simulink library "mbdriLib"  (R2023b)
settings: Solver=ode45  StartTime=0.0  StopTime=10.0  RelTol=1e-3  EnableMultiTasking=on
undefined symbols (not defined in the file): ap, Newton, Raphson, uavParam
libraries: aerolibconvert2 x1, slpidlib x1, sharedtransform x1, $bdroot x1, simulink x1
settings Model: Creator=The MathWorks, Inc.  LastModifiedBy=The MathWorks, Inc.
settings SolverCC: AlgebraicLoopSolver=TrustRegion
settings DataIOCC: LimitDataPoints=on  ReturnWorkspaceOutputs=off
settings OptimizationCC: LifeSpan=inf
settings DebuggingCC: UnconnectedInputMsg=warning  UnconnectedOutputMsg=warning  UnconnectedLineMsg=warning  AllowSymbolicDim=off  SFUnexpectedBacktrackingDiag=warning  SFNoUnconditionalDefaultTransitionDiag=warning  SFExecutionAtInitializationDiag=none  ArithmeticOperatorsInVariantConditions=warning
settings ModelReferenceCC: EnableRefExpFcnMdlSchedulingChecks=on
settings SFSimCC: SimUseLocalCustomCode=off  CustomCodeUndefinedFunction=UseInterfaceOnly
settings RTWCC: RTWUseLocalCustomCode=off  DLArmComputeVersion=19.05
settings CodeAppCC: StateflowObjectComments=on
settings GRTTargetCC: TargetLangStandard=C89/C90 (ANSI)
settings ConfigComp: CovMetricSettings=dw  CovSaveCumulativeToWorkspaceVar=on  CovSaveSingleToWorkspaceVar=on  CovExternalEMLEnable=off

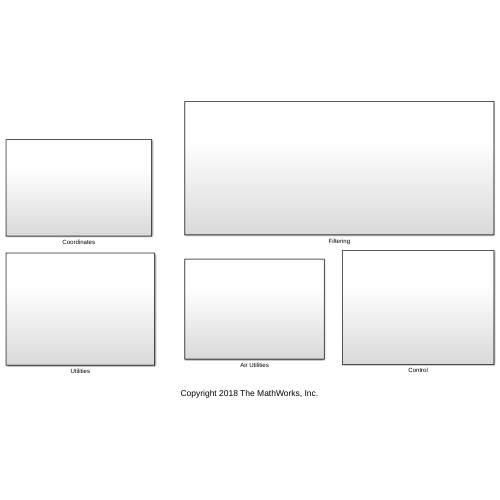
[thumbnail: Simulink's stored preview of the top-level diagram]
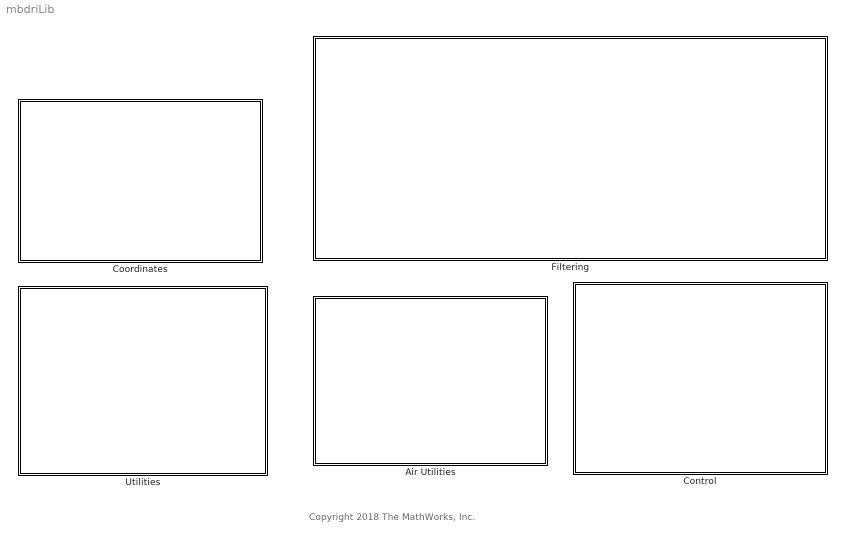
== system mbdriLib ==
  note: Copyright 2018 The MathWorks, Inc.
  Air Utilities : Subsystem
  Control : Subsystem
  Coordinates : Subsystem
  Filtering : Subsystem
  Utilities : Subsystem

== system mbdriLib/Air Utilities ==
  Air Density from Height : Subsystem
  Compute Airspeed : Subsystem

== system mbdriLib/Control ==
  PID Controller : Subsystem  mask(PID){Tsample=0.01, Ndelay=5, upperSaturationLimit=100, lowerSaturationLimit=-100}
      mask prompts: Tsample "Sample Time"; Ndelay "Integer delays for de/dt"; upperSaturationLimit "Upper Saturation Limit"; lowerSaturationLimit "Lower Saturation Limit"
      mask help: PID controller block with anti-windup and saturation limits. Implemented as a discrete forwardl integration which stops integrating when the output is saturated. Derivative is implemented as a numerical derivative with N integer delays to smooth output.
      mask Display:
      | disp('PID')
      | port_label('input',1,'error')
      | port_label('input',3,'gains')
      | port_label('input',2,'reset')
      | port_label('output',1,'output')

== system mbdriLib/Coordinates ==
  RL2B : Subsystem

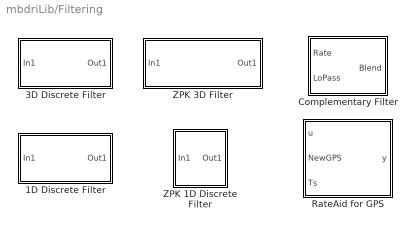
== system mbdriLib/Filtering ==
  1D Discrete Filter : Subsystem  RTWFcnName=TustinFilter3D  mask{bw=40, TSample=0.01}
      mask prompts: bw "Bandwith (Hz)"; TSample "Sample Time"
      mask init:
      | tau = 1/(2*pi*bw);
      | zval = [];
      | pval = -1/tau;
      | kval = 1/tau;
      | 
      | set_param(gcb,'AttributesFormatString', ['Fc = ' num2str(bw)]);
      settings: AttributesFormatString=Fc = 40  RTWFcnNameOpts=User specified  RTWFileNameOpts=Use function name
      mask Display:
      | droots(zval,pval,kval)
      | port_label('input',1,'1D')
  3D Discrete Filter : Subsystem  RTWFcnName=TustinFilter3D  mask{bw=40, TSample=0.01}
      mask prompts: bw "Bandwith (Hz)"; TSample "Sample Time"
      mask init:
      | tau = 1/(2*pi*bw);
      | zval = [];
      | pval = -1/tau;
      | kval = 1/tau;
      | 
      | set_param(gcb,'AttributesFormatString', ['Fc = ' num2str(bw)]);
      settings: AttributesFormatString=Fc = 40  RTWFcnNameOpts=User specified  RTWFileNameOpts=Use function name
      mask Display:
      | droots(zval,pval,kval)
      | port_label('input',1,'3D')
  Complementary Filter : Subsystem  mask{omega=20, T=0.01}
      mask prompts: omega "Cutoff Freq (rad/sec)"; T "Sample Time"
  RateAid for GPS : MATLAB Function  TreatAsAtomicUnit=on
  ZPK 1D Discrete Filter : Subsystem  RTWFcnName=TustinFilter3D  mask{zval=[], pval=[0], kval=1, TSample=0.01}
      mask prompts: zval "Zeros"; pval "Poles"; kval "Gains"; TSample "Sample Time"
      settings: RTWFcnNameOpts=User specified  RTWFileNameOpts=Use function name
      mask Display:
      | droots(zval,pval,kval)
      | port_label('input',1,'1D')
  ZPK 3D Filter : Subsystem  RTWFcnName=TustinFilter3D  mask{zval=[], pval=-1/20, kval=1, TSample=0.01}
      mask prompts: zval "Zeros"; pval "Poles"; kval "Gains"; TSample "Sample Time"
      settings: RTWFcnNameOpts=User specified  RTWFileNameOpts=Use function name
      mask Display:
      | droots(zval,pval,kval)
      | port_label('input',1,'3D')

== system mbdriLib/Utilities ==
  NaiveNoiseGen : Subsystem  mask{np=[0.0005], st=ap.apSampleTime, ng=0.2, ns=[1387]}
      mask prompts: np "Noise Power"; st "Sample Time"; ng "Noise Gain"; ns "Noise Seed"
  Sample GPS data : Subsystem
  yaw rate fact : Subsystem

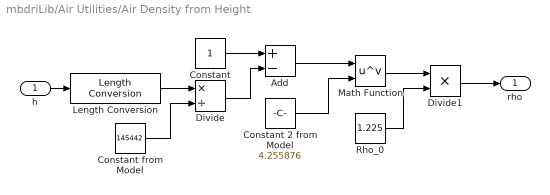
== system mbdriLib/Air Utilities/Air Density from Height ==
  h : Inport  Unit=m
  Add : Sum  Inputs=+-
  Constant : Constant  OutDataTypeStr=single
      settings: AttributesFormatString=%<Value>
  Constant 2 from Model : Constant  Value=4.255876  OutDataTypeStr=single
      settings: AttributesFormatString=%<Value>
  Constant from Model : Constant  Value=145442  OutDataTypeStr=single
      settings: AttributesFormatString=%<Value>
  Divide : Product  Inputs=*/  SampleTime=.01
  Divide1 : Product
  Length Conversion : aerolibconvert2/Length Conversion  IU=m  OU=ft
  Math Function : Math  Operator=pow  SignedPower=on
  Rho_0 : Constant  Description=(Kg/m^3)  Value=1.225  OutDataTypeStr=single
      settings: AttributesFormatString=%<Value>
  "rho " : Outport  Unit=kg/m^3  VectorParamsAs1DForOutWhenUnconnected=off
  wires:
  Constant/1 -> Add/1
  Divide/1 -> Add/2
  h/1 -> Length Conversion/1
  Constant from Model/1 -> Divide/2
  Rho_0/1 -> Divide1/2
  Divide1/1 -> "rho "/1
  Length Conversion/1 -> Divide/1
  Add/1 -> Math Function/1
  Constant 2 from Model/1 -> Math Function/2
  Math Function/1 -> Divide1/1

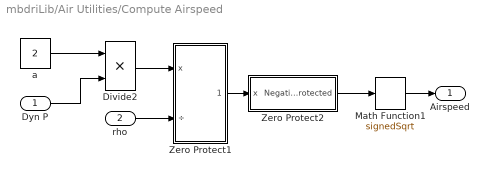
== system mbdriLib/Air Utilities/Compute Airspeed ==
  Dyn P : Inport  Unit=Pa
  rho : Inport  Port=2  Unit=kg/m^3
  Divide2 : Product  SampleTime=.01
  Math Function1 : Sqrt  Operator=signedSqrt  AlgorithmType=Newton-Raphson
  Zero Protect1 : Subsystem
      mask Display:
      | disp('Zero\n Protected\nDivision')
      | port_label('input',1,'x')
      | port_label('input',2,'÷')
  Zero Protect2 : Subsystem
      mask Display:
      | disp('Negative\n Protection')
      | port_label('input',1,'u')
      | port_label('output',1,'y')
  a : Constant  Value=2  OutDataTypeStr=single
      settings: AttributesFormatString=%<Value>
  "Airspeed " : Outport  Unit=m/s  VectorParamsAs1DForOutWhenUnconnected=off
  wires:
  Dyn P/1 -> Divide2/2
  a/1 -> Divide2/1
  Zero Protect2/1(Negative Protected) -> Math Function1/1
  Math Function1/1 -> "Airspeed "/1
  Divide2/1 -> Zero Protect1/1(x)
  rho/1 -> Zero Protect1/2(÷)
  Zero Protect1/1(Zero Protected) -> Zero Protect2/1(x)

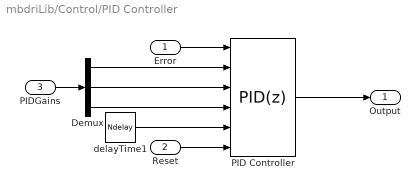
== system mbdriLib/Control/PID Controller ==
  Error : Inport
  Reset : Inport  Port=2
  PIDGains : Inport  Port=3
  Demux : Demux  Outputs=3
  PID Controller : slpidlib/PID Controller  Controller=PID  Form=Parallel  TimeDomain=Discrete-time  UseExternalTs=off  SampleTime=Tsample  IntegratorMethod=Trapezoidal  FilterMethod=Forward Euler  ControllerParametersSource=external  P=1  I=1  UseKiTs=off  D=0  N=100  UseFilter=on  TunerSelectOption=Transfer Function Based (PID Tuner App)  InitialConditionSource=internal  InitialConditionForIntegrator=0  InitialConditionForFilter=0  DifferentiatorICPrevScaledInput=0  ExternalReset=level  TrackingMode=off  Kt=1  LimitOutput=on  SatLimitsSource=internal  UpperSaturationLimit=upperSaturationLimit  LowerSaturationLimit=lowerSaturationLimit  LinearizeAsGain=on  AntiWindupMode=clamping  Kb=1  LimitIntegrator=off  UpperIntegratorSaturationLimit=inf  LowerIntegratorSaturationLimit=-inf  POutMin=[]  POutMax=[]  IOutMin=[]  IOutMax=[]  DOutMin=[]  DOutMax=[]  NOutMin=[]  NOutMax=[]  SumOutMin=[]  SumOutMax=[]  SaturationOutMin=[]  SaturationOutMax=[]  PParamMin=[]  PParamMax=[]  IParamMin=[]  IParamMax=[]  DParamMin=[]  DParamMax=[]  NParamMin=[]  NParamMax=[]  KbParamMin=[]  KbParamMax=[]  KtParamMin=[]  KtParamMax=[]  KbOutMin=[]  KbOutMax=[]  KtOutMin=[]  KtOutMax=[]  IntegratorOutMin=[]  IntegratorOutMax=[]  FilterOutMin=[]  FilterOutMax=[]  SumI1OutMin=[]  SumI1OutMax=[]  SumI2OutMin=[]  SumI2OutMax=[]  SumI3OutMin=[]  SumI3OutMax=[]  SumI4OutMin=[]  SumI4OutMax=[]  SumDOutMin=[]  SumDOutMax=[]  DifferentiatorOutMin=[]  DifferentiatorOutMax=[]  FilterDiffOutCoefMin=[]  FilterDiffOutCoefMax=[]  ReciprocalOutMin=[]  ReciprocalOutMax=[]  SumDenOutMin=[]  SumDenOutMax=[]  SumNumOutMin=[]  SumNumOutMax=[]  DivideOutMin=[]  DivideOutMax=[]  UdiffTsProdOutMin=[]  UdiffTsProdOutMax=[]  NTsProdOutMin=[]  NTsProdOutMax=[]  UintegralTsProdOutMin=[]  UintegralTsProdOutMax=[]  UngainTsProdOutMin=[]  UngainTsProdOutMax=[]  ClampingZeroOutDataTypeStr=Inherit: Inherit via back propagation  ClampingZeroOutMin=[]  ClampingZeroOutMax=[]  FilterDenConstantOutDataTypeStr=Inherit: Inherit via back propagation  FilterDenConstantOutMin=[]  FilterDenConstantOutMax=[]  PCopyOutDataTypeStr=Inherit: Inherit via back propagation  PCopyOutMin=[]  PCopyOutMax=[]  NCopyOutDataTypeStr=Inherit: Inherit via back propagation  NCopyOutMin=[]  NCopyOutMax=[]  IntegratorContinuousStateAttributes=''  IntegratorStateMustResolveToSignalObject=off  IntegratorRTWStateStorageClass=Auto  FilterContinuousStateAttributes=''  FilterStateMustResolveToSignalObject=off  FilterRTWStateStorageClass=Auto  ParallelPVariant=ExternalParameters  IdealPVariant=Disabled  IVariant=ExternalParameters  DVariant=ExternalParameters  IntegratorVariant=Discrete  SatVariant=Enabled  AWVariant=DiscClampingParallel  PCopyVariant=Disabled  TRVariant=Disabled  FdbkBlocksVariant=Feedback  IdealPFdbkVariant=Passthrough  SatFdbkVariant=Passthrough  DerivativeFilterVariant=ForwardEulerFilter  NVariant=ExternalParameters  NCopyVariant=Disabled  FilterICVariant=InternalICsFilter  IntegratorICVariant=InternalICs  ExternalResetVariant=ExternalReset  TRSumVariant=Passthrough  SumFdbkVariant=Enabled  SumVariant=Sum_PID  TsampFilterVariant=InternalTs  TsampNgainVariant=Passthrough  TsampIntegralVariant=Disabled_SignalSpec  ExternalSaturationOutDataTypeStr=Inherit: Same as second input
  delayTime1 : Constant  Value=Ndelay  OutDataTypeStr=single
      settings: AttributesFormatString=%<Value>
  Output : Outport  VectorParamsAs1DForOutWhenUnconnected=off
  wires:
  PIDGains/1 -> Demux/1
  Demux/1 -> PID Controller/2
  Demux/2 -> PID Controller/3
  Demux/3 -> PID Controller/4
  delayTime1/1 -> PID Controller/5
  Reset/1 -> PID Controller/6
  PID Controller/1 -> Output/1
  Error/1 -> PID Controller/1

== system mbdriLib/Coordinates/RL2B ==
  Euler : Inport
  Rotation Angles to Direction Cosine Matrix : sharedtransform/Rotation Angles to Direction Cosine Matrix  rotationOrder=ZYX  aMode=aMode
  Selector : Selector  InputPortWidth=3  IndexOptions=Index vector (dialog)  Indices=[3 2 1]  OutputSizes=1
  RL2B : Outport  VectorParamsAs1DForOutWhenUnconnected=off
  wires:
  Selector/1 -> Rotation Angles to Direction Cosine Matrix/1
  Euler/1 -> Selector/1
  Rotation Angles to Direction Cosine Matrix/1 -> RL2B/1

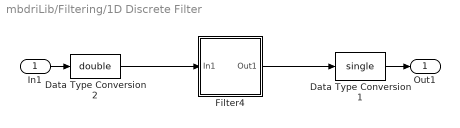
== system mbdriLib/Filtering/1D Discrete Filter ==
  In1 : Inport
  Data Type Conversion1 : DataTypeConversion  OutDataTypeStr=single  SaturateOnIntegerOverflow=off  RndMeth=Floor
  Data Type Conversion2 : DataTypeConversion  OutDataTypeStr=double  SaturateOnIntegerOverflow=off  RndMeth=Floor
  Filter4 : Subsystem  mask{Zeros=zval, Poles=pval, Gain=kval, AbsTol=auto, SampleTime=TSample, method=tustin, Wc=1}
      mask prompts: Zeros "Zeros (enter in s-main:)"; Poles "Poles (enter in s-domain:)"; Gain "Gain (enter in s-domain:)"; AbsTol "Absolute tolerance:"; SampleTime "Sample time:"; Wc "Critical Frequency (Hz):"
      mask init:
      | H = zpk(Zeros, Poles, Gain);
      | Hd = c2d(H, SampleTime, 'tustin');
      | [z, p, g] = zpkdata(Hd);
      | z_d = z{:};
      | p_d = p{:};
      | g_d = g;
      mask TypeOptions method: zoh | foh | tustin | prewarp | matched
      mask Display: droots(Zeros,Poles,Gain)
  Out1 : Outport  VectorParamsAs1DForOutWhenUnconnected=off
  wires:
  Data Type Conversion1/1 -> Out1/1
  In1/1 -> Data Type Conversion2/1
  Data Type Conversion2/1 -> Filter4/1(In1)
  Filter4/1(Out1) -> Data Type Conversion1/1

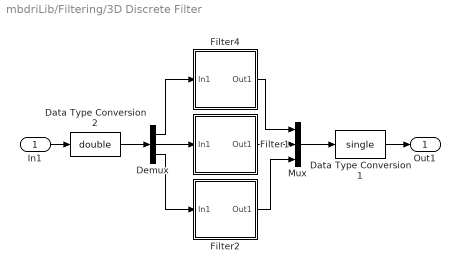
== system mbdriLib/Filtering/3D Discrete Filter ==
  In1 : Inport
  Data Type Conversion1 : DataTypeConversion  OutDataTypeStr=single  SaturateOnIntegerOverflow=off  RndMeth=Floor
  Data Type Conversion2 : DataTypeConversion  OutDataTypeStr=double  SaturateOnIntegerOverflow=off  RndMeth=Floor
  Demux : Demux  Outputs=3
  Filter1 : Subsystem  mask{Zeros=zval, Poles=pval, Gain=kval, AbsTol=auto, SampleTime=TSample, method=tustin, Wc=1}
      mask prompts: Zeros "Zeros (enter in s-main:)"; Poles "Poles (enter in s-domain:)"; Gain "Gain (enter in s-domain:)"; AbsTol "Absolute tolerance:"; SampleTime "Sample time:"; Wc "Critical Frequency (Hz):"
      mask init:
      | H = zpk(Zeros, Poles, Gain);
      | Hd = c2d(H, SampleTime, 'tustin');
      | [z, p, g] = zpkdata(Hd);
      | z_d = z{:};
      | p_d = p{:};
      | g_d = g;
      mask TypeOptions method: zoh | foh | tustin | prewarp | matched
      mask Display: droots(Zeros,Poles,Gain)
  Filter2 : Subsystem  mask{Zeros=zval, Poles=pval, Gain=kval, AbsTol=auto, SampleTime=TSample, method=tustin, Wc=1}
      mask prompts: Zeros "Zeros (enter in s-main:)"; Poles "Poles (enter in s-domain:)"; Gain "Gain (enter in s-domain:)"; AbsTol "Absolute tolerance:"; SampleTime "Sample time:"; Wc "Critical Frequency (Hz):"
      mask init:
      | H = zpk(Zeros, Poles, Gain);
      | Hd = c2d(H, SampleTime, 'tustin');
      | [z, p, g] = zpkdata(Hd);
      | z_d = z{:};
      | p_d = p{:};
      | g_d = g;
      mask TypeOptions method: zoh | foh | tustin | prewarp | matched
      mask Display: droots(Zeros,Poles,Gain)
  Filter4 : Subsystem  mask{Zeros=zval, Poles=pval, Gain=kval, AbsTol=auto, SampleTime=TSample, method=tustin, Wc=1}
      mask prompts: Zeros "Zeros (enter in s-main:)"; Poles "Poles (enter in s-domain:)"; Gain "Gain (enter in s-domain:)"; AbsTol "Absolute tolerance:"; SampleTime "Sample time:"; Wc "Critical Frequency (Hz):"
      mask init:
      | H = zpk(Zeros, Poles, Gain);
      | Hd = c2d(H, SampleTime, 'tustin');
      | [z, p, g] = zpkdata(Hd);
      | z_d = z{:};
      | p_d = p{:};
      | g_d = g;
      mask TypeOptions method: zoh | foh | tustin | prewarp | matched
      mask Display: droots(Zeros,Poles,Gain)
  Mux : Mux  Inputs=3
  Out1 : Outport  VectorParamsAs1DForOutWhenUnconnected=off
  wires:
  Mux/1 -> Data Type Conversion1/1
  In1/1 -> Data Type Conversion2/1
  Filter2/1(Out1) -> Mux/3
  Filter1/1(Out1) -> Mux/2
  Filter4/1(Out1) -> Mux/1
  Demux/3 -> Filter2/1(In1)
  Demux/2 -> Filter1/1(In1)
  Demux/1 -> Filter4/1(In1)
  Data Type Conversion2/1 -> Demux/1
  Data Type Conversion1/1 -> Out1/1

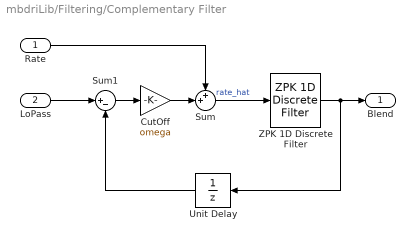
== system mbdriLib/Filtering/Complementary Filter ==
  Rate : Inport
  LoPass : Inport  Port=2
  CutOff : Gain  Gain=omega
      settings: AttributesFormatString=%<Gain>
  Sum : Sum  Inputs=++|
  Sum1 : Sum  Inputs=|+-
  Unit Delay : UnitDelay  SampleTime=ap.apSampleTime  HasFrameUpgradeWarning=on
  ZPK 1D Discrete Filter : $bdroot/Filtering/ZPK 1D Discrete Filter  zval=[]  pval=[0]  kval=1  TSample=ap.apSampleTime
  Blend : Outport  VectorParamsAs1DForOutWhenUnconnected=off
  wires:
  ZPK 1D Discrete Filter/1 -> Blend/1, Unit Delay/1
  Sum/1 -> ZPK 1D Discrete Filter/1  "rate_hat"
  Rate/1 -> Sum/1
  CutOff/1 -> Sum/2
  Sum1/1 -> CutOff/1
  LoPass/1 -> Sum1/1
  Unit Delay/1 -> Sum1/2

== system mbdriLib/Filtering/ZPK 1D Discrete Filter ==
  In1 : Inport
  Filter2 : Subsystem  mask{Zeros=zval, Poles=pval, Gain=kval, AbsTol=auto, SampleTime=TSample, method=tustin, Wc=1}
      mask prompts: Zeros "Zeros (enter in s-main:)"; Poles "Poles (enter in s-domain:)"; Gain "Gain (enter in s-domain:)"; AbsTol "Absolute tolerance:"; SampleTime "Sample time:"; Wc "Critical Frequency (Hz):"
      mask init:
      | H = zpk(Zeros, Poles, Gain);
      | Hd = c2d(H, SampleTime, 'tustin');
      | [z, p, g] = zpkdata(Hd);
      | z_d = z{:};
      | p_d = p{:};
      | g_d = g;
      mask TypeOptions method: zoh | foh | tustin | prewarp | matched
      mask Display: droots(Zeros,Poles,Gain)
  Out1 : Outport  VectorParamsAs1DForOutWhenUnconnected=off
  wires:
  In1/1 -> Filter2/1(In1)
  Filter2/1(Out1) -> Out1/1

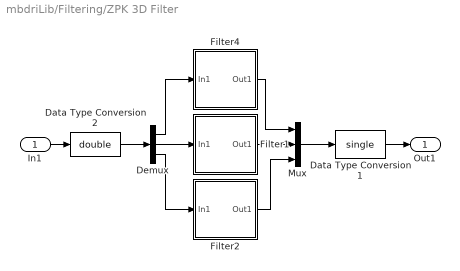
== system mbdriLib/Filtering/ZPK 3D Filter ==
  In1 : Inport
  Data Type Conversion1 : DataTypeConversion  OutDataTypeStr=single  SaturateOnIntegerOverflow=off  RndMeth=Floor
  Data Type Conversion2 : DataTypeConversion  OutDataTypeStr=double  SaturateOnIntegerOverflow=off  RndMeth=Floor
  Demux : Demux  Outputs=3
  Filter1 : Subsystem  mask{Zeros=zval, Poles=pval, Gain=kval, AbsTol=auto, SampleTime=TSample, method=tustin, Wc=1}
      mask prompts: Zeros "Zeros (enter in s-main:)"; Poles "Poles (enter in s-domain:)"; Gain "Gain (enter in s-domain:)"; AbsTol "Absolute tolerance:"; SampleTime "Sample time:"; Wc "Critical Frequency (Hz):"
      mask init:
      | H = zpk(Zeros, Poles, Gain);
      | Hd = c2d(H, SampleTime, 'tustin');
      | [z, p, g] = zpkdata(Hd);
      | z_d = z{:};
      | p_d = p{:};
      | g_d = g;
      mask TypeOptions method: zoh | foh | tustin | prewarp | matched
      mask Display: droots(Zeros,Poles,Gain)
  Filter2 : Subsystem  mask{Zeros=zval, Poles=pval, Gain=kval, AbsTol=auto, SampleTime=TSample, method=tustin, Wc=1}
      mask prompts: Zeros "Zeros (enter in s-main:)"; Poles "Poles (enter in s-domain:)"; Gain "Gain (enter in s-domain:)"; AbsTol "Absolute tolerance:"; SampleTime "Sample time:"; Wc "Critical Frequency (Hz):"
      mask init:
      | H = zpk(Zeros, Poles, Gain);
      | Hd = c2d(H, SampleTime, 'tustin');
      | [z, p, g] = zpkdata(Hd);
      | z_d = z{:};
      | p_d = p{:};
      | g_d = g;
      mask TypeOptions method: zoh | foh | tustin | prewarp | matched
      mask Display: droots(Zeros,Poles,Gain)
  Filter4 : Subsystem  mask{Zeros=zval, Poles=pval, Gain=kval, AbsTol=auto, SampleTime=TSample, method=tustin, Wc=1}
      mask prompts: Zeros "Zeros (enter in s-main:)"; Poles "Poles (enter in s-domain:)"; Gain "Gain (enter in s-domain:)"; AbsTol "Absolute tolerance:"; SampleTime "Sample time:"; Wc "Critical Frequency (Hz):"
      mask init:
      | H = zpk(Zeros, Poles, Gain);
      | Hd = c2d(H, SampleTime, 'tustin');
      | [z, p, g] = zpkdata(Hd);
      | z_d = z{:};
      | p_d = p{:};
      | g_d = g;
      mask TypeOptions method: zoh | foh | tustin | prewarp | matched
      mask Display: droots(Zeros,Poles,Gain)
  Mux : Mux  Inputs=3
  Out1 : Outport  VectorParamsAs1DForOutWhenUnconnected=off
  wires:
  Data Type Conversion1/1 -> Out1/1
  Data Type Conversion2/1 -> Demux/1
  Demux/1 -> Filter4/1(In1)
  Demux/2 -> Filter1/1(In1)
  Demux/3 -> Filter2/1(In1)
  Filter4/1(Out1) -> Mux/1
  Filter1/1(Out1) -> Mux/2
  Filter2/1(Out1) -> Mux/3
  In1/1 -> Data Type Conversion2/1
  Mux/1 -> Data Type Conversion1/1

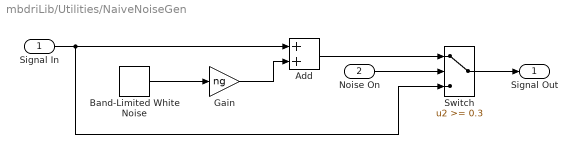
== system mbdriLib/Utilities/NaiveNoiseGen ==
  Signal In : Inport
  Noise On : Inport  Port=2
  Add : Sum
  Band-Limited White Noise : simulink/Sources/Band-Limited White Noise  Cov=np  Ts=st  seed=ns
  Gain : Gain  Gain=ng
      settings: AttributesFormatString=%<Gain>
  Switch : Switch  Threshold=0.3  SaturateOnIntegerOverflow=off  InputSameDT=off
  Signal Out : Outport  VectorParamsAs1DForOutWhenUnconnected=off
  wires:
  Band-Limited White Noise/1 -> Gain/1
  Add/1 -> Switch/1
  Noise On/1 -> Switch/2
  Switch/1 -> Signal Out/1
  Signal In/1 -> Switch/3, Add/1
  Gain/1 -> Add/2

== system mbdriLib/Utilities/Sample GPS data ==
  GPS : Inport
  Rate Transition : RateTransition  OutPortSampleTime=sensors.gpsRefreshRate
      settings: AttributesFormatString=%<OutPortSampleTime>
  GPS_samp : Outport  VectorParamsAs1DForOutWhenUnconnected=off
  wires:
  GPS/1 -> Rate Transition/1
  Rate Transition/1 -> GPS_samp/1

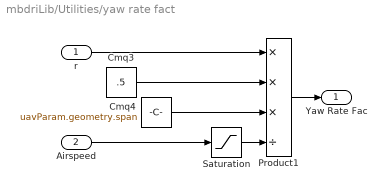
== system mbdriLib/Utilities/yaw rate fact ==
  r : Inport
  Airspeed : Inport  Port=2
  Cmq3 : Constant  Value=.5
      settings: AttributesFormatString=%<Value>
  Cmq4 : Constant  Value=uavParam.geometry.span
      settings: AttributesFormatString=%<Value>
  Product1 : Product  Inputs=***/  SaturateOnIntegerOverflow=on  OutDataTypeStr=Inherit: Same as first input
  Saturation : Saturate  UpperLimit=inf  LowerLimit=0.1
      settings: AttributesFormatString="[%<LowerLimit>  %<UpperLimit>]"
  Yaw Rate Fac : Outport  VectorParamsAs1DForOutWhenUnconnected=off
  wires:
  Saturation/1 -> Product1/4
  Airspeed/1 -> Saturation/1
  Cmq4/1 -> Product1/3
  Cmq3/1 -> Product1/2
  r/1 -> Product1/1
  Product1/1 -> Yaw Rate Fac/1

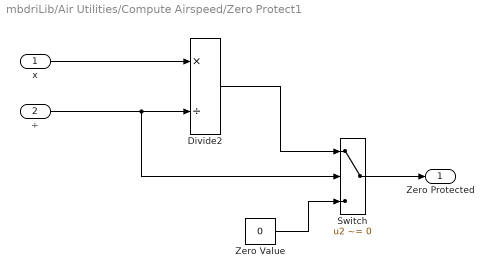
== system mbdriLib/Air Utilities/Compute Airspeed/Zero Protect1 ==
  x : Inport
  ÷ : Inport  Port=2
  Divide2 : Product  Inputs=*/
  Switch : Switch  Criteria=u2 ~= 0  Threshold=0.1  OutDataTypeStr=Inherit: Inherit via back propagation  SaturateOnIntegerOverflow=off  InputSameDT=off
  Zero Value : Constant  Value=0  OutDataTypeStr=single
  Zero Protected : Outport  VectorParamsAs1DForOutWhenUnconnected=off
  wires:
  ÷/1 -> Switch/2, Divide2/2
  Zero Value/1 -> Switch/3
  Switch/1 -> Zero Protected/1
  Divide2/1 -> Switch/1
  x/1 -> Divide2/1

== system mbdriLib/Air Utilities/Compute Airspeed/Zero Protect2 ==
  x : Inport
  Switch : Switch  OutDataTypeStr=Inherit: Inherit via back propagation  SaturateOnIntegerOverflow=off  InputSameDT=off
  Zero Value : Constant  Value=0  OutDataTypeStr=single
  Negative Protected : Outport  VectorParamsAs1DForOutWhenUnconnected=off
  wires:
  x/1 -> Switch/2, Switch/1
  Switch/1 -> Negative Protected/1
  Zero Value/1 -> Switch/3

== system mbdriLib/Filtering/1D Discrete Filter/Filter4 ==
  In1 : Inport
  Discrete Zero-Pole : DiscreteZeroPole  Zeros=z_d  Poles=p_d  Gain=g_d  SampleTime=-1
  Out1 : Outport  VectorParamsAs1DForOutWhenUnconnected=off
  wires:
  Discrete Zero-Pole/1 -> Out1/1
  In1/1 -> Discrete Zero-Pole/1

== system mbdriLib/Filtering/3D Discrete Filter/Filter1 ==
  In1 : Inport
  Discrete Zero-Pole : DiscreteZeroPole  Zeros=z_d  Poles=p_d  Gain=g_d  SampleTime=-1
  Out1 : Outport  VectorParamsAs1DForOutWhenUnconnected=off
  wires:
  Discrete Zero-Pole/1 -> Out1/1
  In1/1 -> Discrete Zero-Pole/1

== system mbdriLib/Filtering/3D Discrete Filter/Filter2 ==
  In1 : Inport
  Discrete Zero-Pole : DiscreteZeroPole  Zeros=z_d  Poles=p_d  Gain=g_d  SampleTime=-1
  Out1 : Outport  VectorParamsAs1DForOutWhenUnconnected=off
  wires:
  In1/1 -> Discrete Zero-Pole/1
  Discrete Zero-Pole/1 -> Out1/1

== system mbdriLib/Filtering/3D Discrete Filter/Filter4 ==
  In1 : Inport
  Discrete Zero-Pole : DiscreteZeroPole  Zeros=z_d  Poles=p_d  Gain=g_d  SampleTime=-1
  Out1 : Outport  VectorParamsAs1DForOutWhenUnconnected=off
  wires:
  In1/1 -> Discrete Zero-Pole/1
  Discrete Zero-Pole/1 -> Out1/1

== system mbdriLib/Filtering/ZPK 1D Discrete Filter/Filter2 ==
  In1 : Inport
  Discrete Zero-Pole : DiscreteZeroPole  Zeros=z_d  Poles=p_d  Gain=g_d  SampleTime=-1
  Out1 : Outport  VectorParamsAs1DForOutWhenUnconnected=off
  wires:
  In1/1 -> Discrete Zero-Pole/1
  Discrete Zero-Pole/1 -> Out1/1

== system mbdriLib/Filtering/ZPK 3D Filter/Filter1 ==
  In1 : Inport
  Discrete Zero-Pole : DiscreteZeroPole  Zeros=z_d  Poles=p_d  Gain=g_d  SampleTime=-1
  Out1 : Outport  VectorParamsAs1DForOutWhenUnconnected=off
  wires:
  In1/1 -> Discrete Zero-Pole/1
  Discrete Zero-Pole/1 -> Out1/1

== system mbdriLib/Filtering/ZPK 3D Filter/Filter2 ==
  In1 : Inport
  Discrete Zero-Pole : DiscreteZeroPole  Zeros=z_d  Poles=p_d  Gain=g_d  SampleTime=-1
  Out1 : Outport  VectorParamsAs1DForOutWhenUnconnected=off
  wires:
  Discrete Zero-Pole/1 -> Out1/1
  In1/1 -> Discrete Zero-Pole/1

== system mbdriLib/Filtering/ZPK 3D Filter/Filter4 ==
  In1 : Inport
  Discrete Zero-Pole : DiscreteZeroPole  Zeros=z_d  Poles=p_d  Gain=g_d  SampleTime=-1
  Out1 : Outport  VectorParamsAs1DForOutWhenUnconnected=off
  wires:
  Discrete Zero-Pole/1 -> Out1/1
  In1/1 -> Discrete Zero-Pole/1

== matlab function mbdriLib/Filtering/RateAid for GPS ==
  data: u input size=1; y output size=1; NewGPS input size=1; Ts input size=1 =Ts
function y = RateAid(u,NewGPS,Ts)
persistent LastU;
persistent TimeSinceLast;
persistent rate;
persistent OldRate;

if (isempty(LastU))
    LastU = single(0.);
    TimeSinceLast = single(Ts);
    rate = single(0);
    OldRate = single(0);
end

if (NewGPS)
    OldRate = rate;
    rate = single((u - LastU)/TimeSinceLast);
    TimeSinceLast = single(0);
    LastU = u;
end
y = u + ( .5*rate + .5*OldRate )*TimeSinceLast;
TimeSinceLast = TimeSinceLast + Ts;
